simulink model "ssc_p"  (R2014a)
settings: Solver=ode45  StartTime=0.0  StopTime=10.0  RelTol=1e-3
settings Model: Creator=user  LastModifiedBy=Wolfgang
settings SolverCC: ZeroCrossAlgorithm=Adaptive
settings OptimizationCC: SimCompilerOptimization=On
settings DebuggingCC: UnderspecifiedInitializationDetection=Classic  SolverPrmCheckMsg=none

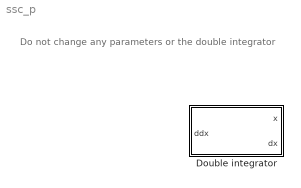
== system ssc_p ==
  note: Do not change any parameters or the double integrator
  Double integrator : Subsystem
      mask Display: dpoly([1],[1 0 0], 's')

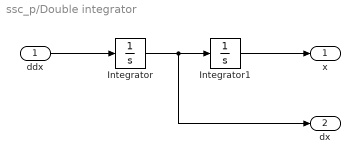
== system ssc_p/Double integrator ==
  ddx : Inport
  Integrator : Integrator
  Integrator1 : Integrator
  x : Outport
  dx : Outport  Port=2
  wires:
  Integrator/1 -> dx/1, Integrator1/1
  Integrator1/1 -> x/1
  ddx/1 -> Integrator/1
